simulink model "verify_alfa_window_in_mdl"  (R2016b)
settings: Solver=VariableStepDiscrete  StartTime=12*3600  StopTime=10+12*3600  MaxStep=1  RelTol=1e-3  EnableMultiTasking=on
libraries: carnot x4, simulink x1
settings Model: Creator=drhf  LastModifiedBy=srrt
settings DataIOCC: SaveFormat=Array  SignalLoggingSaveFormat=ModelDataLogs
settings OptimizationCC: ExpressionDepthLimit=2147483647  LifeSpan=inf
settings DebuggingCC: UnderspecifiedInitializationDetection=Classic  MergeDetectMultiDrivingBlocksExec=none  SolverPrmCheckMsg=warning  FcnCallInpInsideContextMsg=warning  StateNameClashWarn=warning  SFUnexpectedBacktrackingDiag=warning  SFNoUnconditionalDefaultTransitionDiag=warning  SFExecutionAtInitializationDiag=none
settings HardwareCC: ProdBitPerPointer=32  ProdBitPerSizeT=32  ProdBitPerPtrDiffT=32  ProdLargestAtomicFloat=None  ProdIntDivRoundTo=Undefined  ProdEndianess=Unspecified  ProdWordSize=32  ProdHWDeviceType=32-bit Generic
settings ModelReferenceCC: PropagateSignalLabelsOutOfModel=off
settings GRTTargetCC: TargetLangStandard=C89/C90 (ANSI)  GeneratePreprocessorConditionals=Disable all  CombineOutputUpdateFcns=off  GRTInterface=on
settings ConfigComp: CovMetricSettings=dw  CovHtmlReporting=on  CovSaveCumulativeToWorkspaceVar=on  CovSaveSingleToWorkspaceVar=on  CovExternalEMLEnable=off

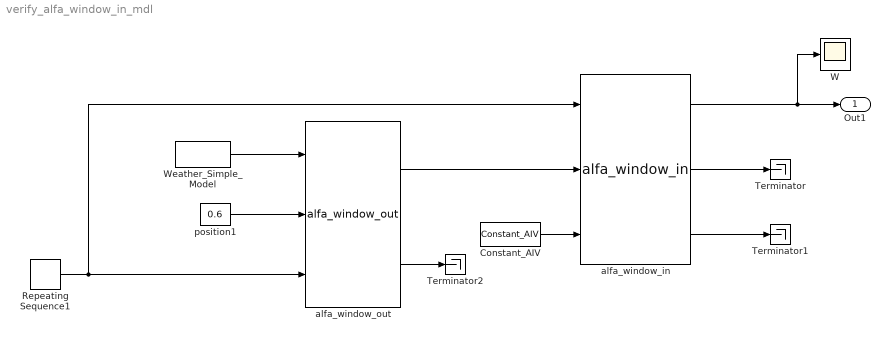
== system verify_alfa_window_in_mdl ==
  Constant_AIV : carnot/Source/Ventilation/Constant_AIV  Tsens=20  Tcon=20  Trad=20  mw=0.012  mco=0.01  rhoair=1.2  cpair=1004  pair=100000  nair=0.5
  Repeating Sequence1 : simulink/Sources/Repeating Sequence  rep_seq_t=[0 10]  rep_seq_y=[10 30]
  Terminator : Terminator
  Terminator1 : Terminator
  Terminator2 : Terminator
  W : Scope
  Weather_Simple_Model : carnot/Weather/Weather_Simple_Model  lat=60  Ibn=900  Idg=100  tamb=5  deltaTsky=-6  rh=50  precip="10e-3/24/3600           % 10 mm in 24 h"  cloud=0.125  p=1013e2  vw=1  wdir=270
  alfa_window_in : carnot/Load/Houses/heat_transfer/alfa_window_in  gvalue=0.7  emission_in=0.87  wallsurface=1  frame=0.1  numlayer=2
  alfa_window_out : carnot/Load/Houses/heat_transfer/alfa_window_out  pos=0  absorption_out=0.01  emission_out=0.87  frame=0.1
  position1 : Constant  Value=0.6
  Out1 : Outport
  wires:
  alfa_window_in/1 -> W/1, Out1/1
  Repeating Sequence1/1 -> alfa_window_in/1, alfa_window_out/3
  Constant_AIV/1 -> alfa_window_in/3
  alfa_window_in/2 -> Terminator/1
  alfa_window_in/3 -> Terminator1/1
  alfa_window_out/1 -> alfa_window_in/2
  Weather_Simple_Model/1 -> alfa_window_out/1
  position1/1 -> alfa_window_out/2
  alfa_window_out/2 -> Terminator2/1
